simulink model "ex2"  (R2023b)
settings: Solver=VariableStepAuto  StartTime=0.0  StopTime=50  RelTol=1e-3
settings Model: Creator=chapo  LastModifiedBy=chapo

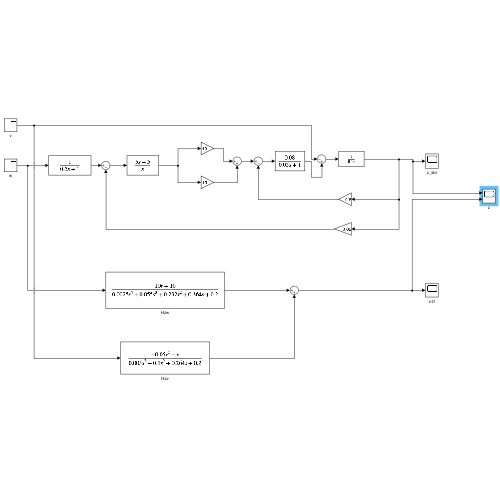
[thumbnail: Simulink's stored preview of the top-level diagram]
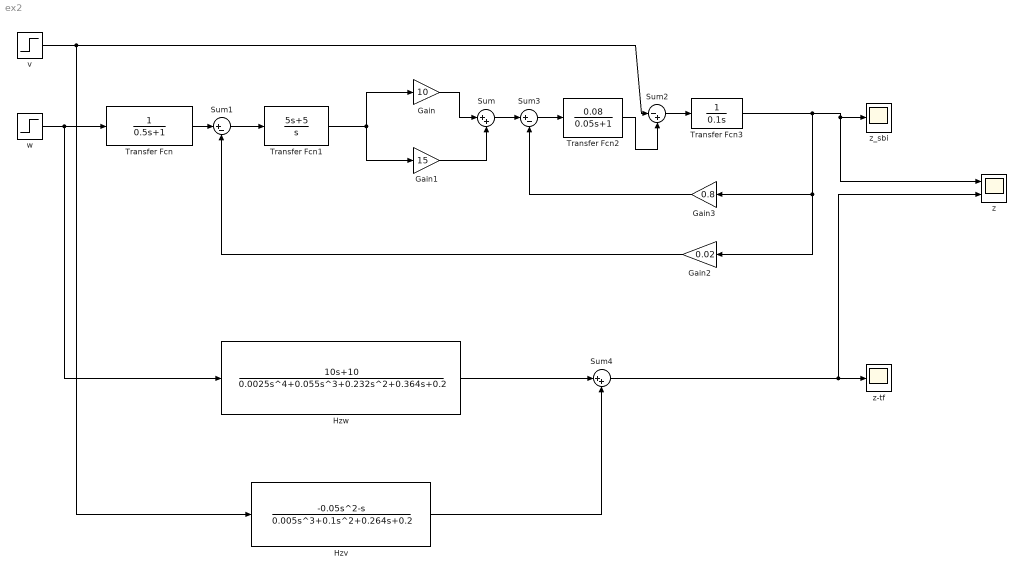
== system ex2 ==
  Gain : Gain  Gain=10
  Gain1 : Gain  Gain=15
  Gain2 : Gain  Gain=0.02
  Gain3 : Gain  Gain=0.8
  Hzv : TransferFcn  Numerator=[-0.05 -1 0]  Denominator=[0.005 0.1 0.264 0.2]
  Hzw : TransferFcn  Numerator=[10 10]  Denominator=[0.0025 0.055 0.232 0.364 0.2]
  Sum : Sum  Inputs=|++
  Sum1 : Sum  Inputs=|+-
  Sum2 : Sum  Inputs=|-+
  Sum3 : Sum  Inputs=|+-
  Sum4 : Sum  Inputs=|++
  Transfer Fcn : TransferFcn  Denominator=[0.5 1]
  Transfer Fcn1 : TransferFcn  Numerator=[5 5]  Denominator=[1 0]
  Transfer Fcn2 : TransferFcn  Numerator=[0.08]  Denominator=[0.05 1]
  Transfer Fcn3 : TransferFcn  Denominator=[0.1 0]
  v : Step  Time=25  SampleTime=0
  w : Step  After=5  SampleTime=0
  z : Scope  NumInputPorts=2
  z-tf : Scope
  z_sbi : Scope
  wires:
  Transfer Fcn1/1 -> Gain1/1, Gain/1
  Gain1/1 -> Sum/2
  Gain/1 -> Sum/1
  Sum2/1 -> Transfer Fcn3/1
  Transfer Fcn3/1 -> Gain2/1, Gain3/1, z/1, z_sbi/1
  Transfer Fcn/1 -> Sum1/1
  Sum1/1 -> Transfer Fcn1/1
  Gain2/1 -> Sum1/2
  w/1 -> Hzw/1, Transfer Fcn/1
  Sum3/1 -> Transfer Fcn2/1
  Sum/1 -> Sum3/1
  Gain3/1 -> Sum3/2
  Transfer Fcn2/1 -> Sum2/2
  v/1 -> Hzv/1, Sum2/1
  Hzw/1 -> Sum4/1
  Hzv/1 -> Sum4/2
  Sum4/1 -> z/2, z-tf/1
